simulink model "mod_1R2011a"  (Simulink 7.7)
settings: Solver=ode45  StartTime=0.0  StopTime=10.0  RelTol=1e-3
settings Model: Creator=Professor Dingyu Xue  LastModifiedBy=Professor Dingyu Xue
settings OptimizationCC: InlineParams=on

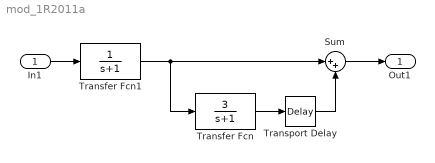
== system mod_1R2011a ==
  In1 : Inport
  Sum : Sum  Inputs=|++
  Transfer Fcn : TransferFcn  Numerator=3  Denominator=[1 1]
  Transfer Fcn1 : TransferFcn  Numerator=1  Denominator=[1 1]
  Transport Delay : TransportDelay
  Out1 : Outport
  wires:
  In1/1 -> Transfer Fcn1/1
  Sum/1 -> Out1/1
  Transfer Fcn/1 -> Transport Delay/1
  Transport Delay/1 -> Sum/2
  Transfer Fcn1/1 -> Sum/1, Transfer Fcn/1
